simulink model "Navigation_KF_Subsystem_child"  (R2016a)
settings: configuration reference "AR_Drone_ConfigSet" (kept outside this file)
undefined symbols (not defined in the file or in its folder): Accel_Calib_Gain, Accel_Calib_Offset, DiscIntNeverNeededParam, Mag_Calib_Gain_Vector, Mag_Calib_Offset_Vector
libraries: aerolibtransform2 x4, vrlib x4
(part 1 of 2)
settings Model: DataDictionary=ArDroneDataDictionary.sldd  SimulationMode=external  Creator=darenlee  LastModifiedBy=sannem
settings ConfigSetRef: DDName=ArDroneDataDictionary.sldd

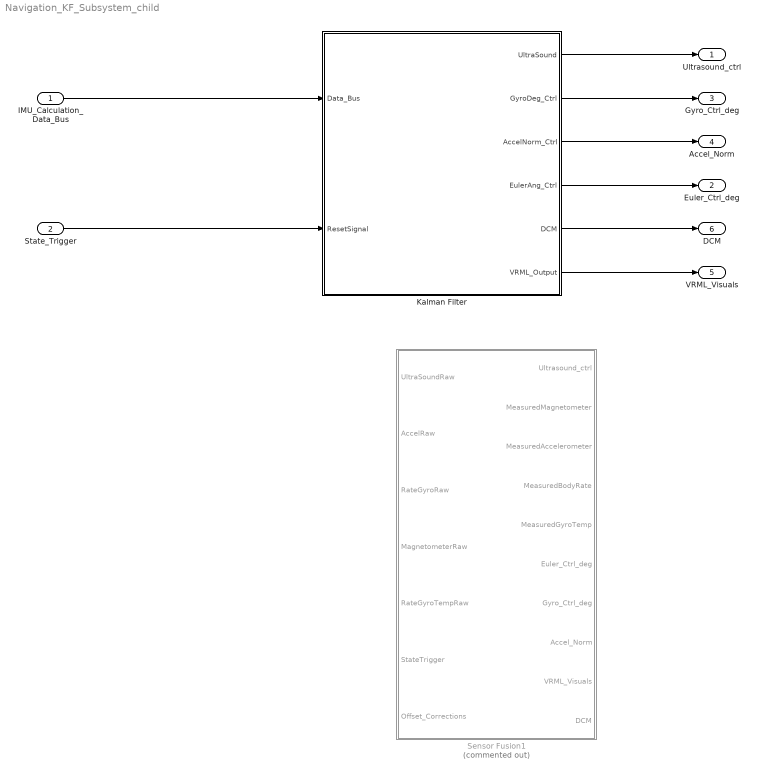
== system Navigation_KF_Subsystem_child ==
  IMU_Calculation_Data_Bus : Inport  OutDataTypeStr=Bus: Measurement_Calculation_Bus
  State_Trigger : Inport  Port=2  OutDataTypeStr=int16
  Kalman Filter : Subsystem
  Sensor Fusion1 : Subsystem  Commented=on
  Ultrasound_ctrl : Outport
  Euler_Ctrl_deg : Outport  Port=2
  Gyro_Ctrl_deg : Outport  Port=3
  Accel_Norm : Outport  Port=4
  VRML_Visuals : Outport  Port=5
  DCM : Outport  Port=6
  wires:
  IMU_Calculation_Data_Bus/1 -> Kalman Filter/1(Data_Bus)
  State_Trigger/1 -> Kalman Filter/2(ResetSignal)
  Kalman Filter/1(UltraSound) -> Ultrasound_ctrl/1
  Kalman Filter/2(GyroDeg_Ctrl) -> Gyro_Ctrl_deg/1
  Kalman Filter/3(AccelNorm_Ctrl) -> Accel_Norm/1
  Kalman Filter/4(EulerAng_Ctrl) -> Euler_Ctrl_deg/1
  Kalman Filter/5(DCM) -> DCM/1
  Kalman Filter/6(VRML_Output) -> VRML_Visuals/1

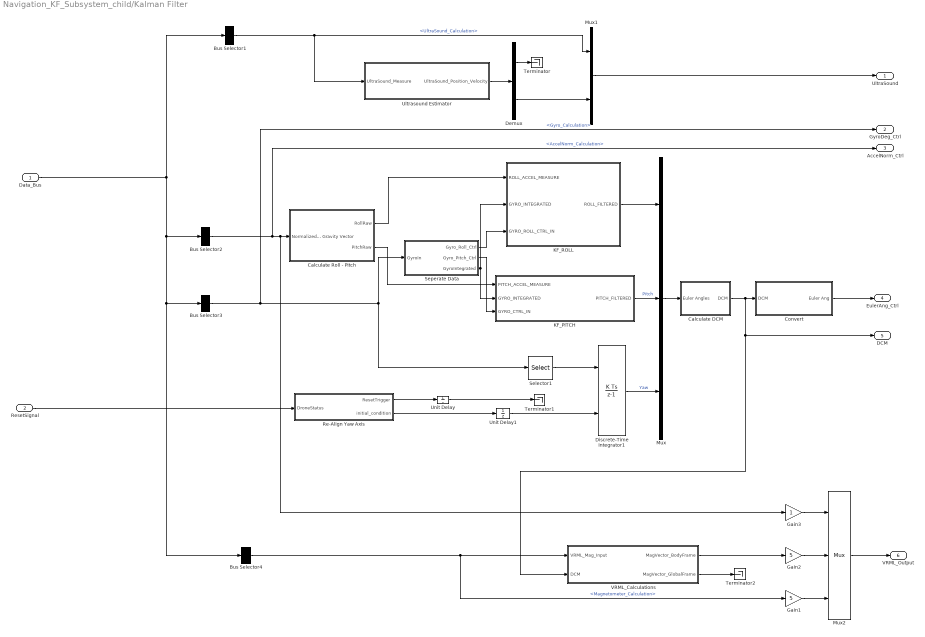
== system Navigation_KF_Subsystem_child/Kalman Filter ==
  Data_Bus : Inport
  ResetSignal : Inport  Port=2
  Bus Selector1 : BusSelector  OutputSignals=UltraSound_Calculation
  Bus Selector2 : BusSelector  OutputSignals=AccelNorm_Calculation
  Bus Selector3 : BusSelector  OutputSignals=Gyro_Calculation
  Bus Selector4 : BusSelector  OutputSignals=Magnetometer_Calculation
  Calculate DCM : Subsystem
  Calculate Roll - Pitch : Subsystem
  Convert : Subsystem
  Demux : Demux  Outputs=2
  Discrete-Time Integrator1 : DiscreteIntegrator  InitialConditionSource=external  SampleTime=1/400  OutDataTypeStr=double  ICPrevOutput=DiscIntNeverNeededParam  ICPrevScaledInput=DiscIntNeverNeededParam
  Gain1 : Gain  Gain=5  OutDataTypeStr=double
  Gain2 : Gain  Gain=5  OutDataTypeStr=double
  Gain3 : Gain  OutDataTypeStr=double
  KF_PITCH : Subsystem
  KF_ROLL : Subsystem
  Mux : Mux  Inputs=3
  Mux1 : Mux  Inputs=2
  Mux2 : Mux  Inputs=3
  Re-Align Yaw Axis : MATLAB Function  TreatAsAtomicUnit=on
  Selector1 : Selector  IndexMode=Zero-based  InputPortWidth=3  IndexOptions=Index vector (dialog)  Indices=[2]  OutputSizes=1
  Seperate Data : Subsystem
  Terminator : Terminator
  Terminator1 : Terminator
  Terminator2 : Terminator
  Ultrasound Estimator : Subsystem
  Unit Delay : UnitDelay  SampleTime=-1
  Unit Delay1 : UnitDelay  SampleTime=-1
  VRML_Calculations : Subsystem
  UltraSound : Outport
  GyroDeg_Ctrl : Outport  Port=2
  AccelNorm_Ctrl : Outport  Port=3
  EulerAng_Ctrl : Outport  Port=4
  DCM : Outport  Port=5
  VRML_Output : Outport  Port=6
  wires:
  Calculate DCM/1(DCM) -> Convert/1(DCM), DCM/1, VRML_Calculations/2(DCM)
  Bus Selector1/1 -> Ultrasound Estimator/1(UltraSound_Measure), Mux1/1  "<UltraSound_Calculation>"
  Unit Delay/1 -> Terminator1/1
  Data_Bus/1 -> Bus Selector4/1, Bus Selector3/1, Bus Selector2/1, Bus Selector1/1
  Re-Align Yaw Axis/1(ResetTrigger) -> Unit Delay/1
  Bus Selector4/1 -> Gain1/1, VRML_Calculations/1(VRML_Mag_Input)  "<Magnetometer_Calculation>"
  Unit Delay1/1 -> Discrete-Time Integrator1/2
  Bus Selector3/1 -> Selector1/1, Seperate Data/1(GyroIn), GyroDeg_Ctrl/1  "<Gyro_Calculation>"
  Calculate Roll - Pitch/2(PitchRaw) -> KF_PITCH/1(PITCH_ACCEL_MEASURE)
  Seperate Data/2(Gyro_Pitch_Ctrl) -> KF_PITCH/3(GYRO_CTRL_IN)
  Discrete-Time Integrator1/1 -> Mux/3  "Yaw"
  Mux/1 -> Calculate DCM/1(Euler Angles)
  Bus Selector2/1 -> Calculate Roll - Pitch/1(Normalized Gravity Vector), Gain3/1, AccelNorm_Ctrl/1  "<AccelNorm_Calculation>"
  Gain3/1 -> Mux2/1
  Ultrasound Estimator/1("UltraSound_Position_Velocity ") -> Demux/1
  KF_PITCH/1(PITCH_FILTERED) -> Mux/2  "Pitch"
  KF_ROLL/1(ROLL_FILTERED) -> Mux/1
  ResetSignal/1 -> Re-Align Yaw Axis/1(DroneStatus)
  Calculate Roll - Pitch/1(RollRaw) -> KF_ROLL/1(ROLL_ACCEL_MEASURE)
  VRML_Calculations/1(MagVector_BodyFrame) -> Gain2/1
  Gain2/1 -> Mux2/2
  Convert/1(Euler Ang) -> EulerAng_Ctrl/1
  Mux2/1 -> VRML_Output/1
  Demux/2 -> Mux1/2
  Gain1/1 -> Mux2/3
  Re-Align Yaw Axis/2(initial_condition) -> Unit Delay1/1
  Mux1/1 -> UltraSound/1
  Seperate Data/3(GyroIntegrated) -> KF_PITCH/2(GYRO_INTEGRATED), KF_ROLL/2(GYRO_INTEGRATED)
  Demux/1 -> Terminator/1
  VRML_Calculations/2(MagVector_GlobalFrame) -> Terminator2/1
  Selector1/1 -> Discrete-Time Integrator1/1
  Seperate Data/1(Gyro_Roll_Ctrl) -> KF_ROLL/3(GYRO_ROLL_CTRL_IN)

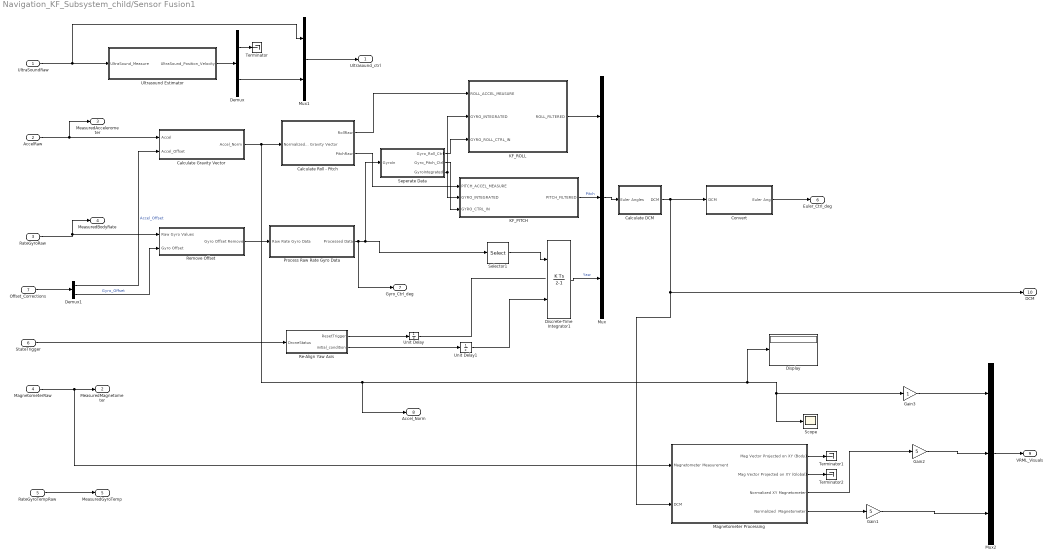
== system Navigation_KF_Subsystem_child/Sensor Fusion1 ==
  UltraSoundRaw : Inport
  AccelRaw : Inport  Port=2
  RateGyroRaw : Inport  Port=3
  MagnetometerRaw : Inport  Port=4
  RateGyroTempRaw : Inport  Port=5
  StateTrigger : Inport  Port=6
  Offset_Corrections : Inport  Port=7
  Calculate DCM : Subsystem
  Calculate Gravity Vector : Subsystem
  Calculate Roll - Pitch : Subsystem
  Convert : Subsystem
  Demux : Demux  Outputs=2
  Demux1 : Demux  Outputs=[2 3]
  Discrete-Time Integrator1 : DiscreteIntegrator  InitialConditionSource=external  SampleTime=1/400  OutDataTypeStr=double  ICPrevOutput=DiscIntNeverNeededParam  ICPrevScaledInput=DiscIntNeverNeededParam
  Display : Display
  Gain1 : Gain  Gain=5  OutDataTypeStr=double
  Gain2 : Gain  Gain=5  OutDataTypeStr=double
  Gain3 : Gain  OutDataTypeStr=double
  KF_PITCH : Subsystem
  KF_ROLL : Subsystem
  Magnetometer Processing : Subsystem  TreatAsAtomicUnit=on
      settings: RTWSystemCode=Inline
  Mux : Mux  Inputs=3
  Mux1 : Mux  Inputs=2
  Mux2 : Mux  Inputs=3
  Process Raw Rate Gyro Data : Subsystem
  Re-Align Yaw Axis : MATLAB Function  TreatAsAtomicUnit=on
  Remove Offset : Subsystem
  Scope : Scope
  Selector1 : Selector  IndexMode=Zero-based  InputPortWidth=3  IndexOptions=Index vector (dialog)  Indices=[2]  OutputSizes=1
  Seperate Data : Subsystem
  Terminator : Terminator
  Terminator1 : Terminator
  Terminator2 : Terminator
  Ultrasound Estimator : Subsystem
  Unit Delay : UnitDelay  SampleTime=-1
  Unit Delay1 : UnitDelay  SampleTime=-1
  Ultrasound_ctrl : Outport
  MeasuredMagnetometer : Outport  Port=2
  MeasuredAccelerometer : Outport  Port=3
  MeasuredBodyRate : Outport  Port=4
  MeasuredGyroTemp : Outport  Port=5
  Euler_Ctrl_deg : Outport  Port=6
  Gyro_Ctrl_deg : Outport  Port=7
  Accel_Norm : Outport  Port=8
  VRML_Visuals : Outport  Port=9
  DCM : Outport  Port=10
  wires:
  Gain1/1 -> Mux2/3
  Gain3/1 -> Mux2/1
  Calculate Roll - Pitch/1(RollRaw) -> KF_ROLL/1(ROLL_ACCEL_MEASURE)
  Calculate Roll - Pitch/2(PitchRaw) -> KF_PITCH/1(PITCH_ACCEL_MEASURE)
  Process Raw Rate Gyro Data/1(Processed Data) -> Selector1/1, Seperate Data/1(GyroIn), Gyro_Ctrl_deg/1
  Mux1/1 -> Ultrasound_ctrl/1
  Ultrasound Estimator/1("UltraSound_Position_Velocity ") -> Demux/1
  Demux/2 -> Mux1/2
  Demux/1 -> Terminator/1
  Discrete-Time Integrator1/1 -> Mux/3  "Yaw"
  KF_PITCH/1(PITCH_FILTERED) -> Mux/2  "Pitch"
  KF_ROLL/1(ROLL_FILTERED) -> Mux/1
  Calculate DCM/1(DCM) -> Magnetometer Processing/2(DCM), DCM/1, Convert/1(DCM)
  Mux/1 -> Calculate DCM/1(Euler Angles)
  Calculate Gravity Vector/1(Accel_Norm) -> Accel_Norm/1, Display/1, Scope/1, Gain3/1, Calculate Roll - Pitch/1(Normalized Gravity Vector)
  Magnetometer Processing/4(Normalized  Magnetometer) -> Gain1/1
  Magnetometer Processing/3(Normalized XY Magnetometer) -> Gain2/1
  Magnetometer Processing/1(Mag Vector Projected on XY (Body)) -> Terminator1/1
  Magnetometer Processing/2(Mag Vector Projected on XY (Global)) -> Terminator2/1
  Remove Offset/1(Gyro Offset Remove) -> Process Raw Rate Gyro Data/1(Raw Rate Gyro Data)
  UltraSoundRaw/1 -> Mux1/1, Ultrasound Estimator/1(UltraSound_Measure)
  MagnetometerRaw/1 -> MeasuredMagnetometer/1, Magnetometer Processing/1(Magnetometer Measurement)
  RateGyroRaw/1 -> MeasuredBodyRate/1, Remove Offset/1(Raw Gyro Values)
  RateGyroTempRaw/1 -> MeasuredGyroTemp/1
  AccelRaw/1 -> MeasuredAccelerometer/1, Calculate Gravity Vector/1(Accel)
  Convert/1(Euler Ang) -> Euler_Ctrl_deg/1
  Re-Align Yaw Axis/1(ResetTrigger) -> Unit Delay/1
  StateTrigger/1 -> Re-Align Yaw Axis/1(DroneStatus)
  Unit Delay/1 -> ?
  Re-Align Yaw Axis/2(initial_condition) -> Unit Delay1/1
  Unit Delay1/1 -> Discrete-Time Integrator1/2
  Selector1/1 -> Discrete-Time Integrator1/1
  Seperate Data/1(Gyro_Roll_Ctrl) -> KF_ROLL/3(GYRO_ROLL_CTRL_IN)
  Seperate Data/2(Gyro_Pitch_Ctrl) -> KF_PITCH/3(GYRO_CTRL_IN)
  Seperate Data/3(GyroIntegrated) -> KF_PITCH/2(GYRO_INTEGRATED), KF_ROLL/2(GYRO_INTEGRATED)
  Offset_Corrections/1 -> Demux1/1
  Demux1/1 -> Calculate Gravity Vector/2(Accel_Offset)  "Accel_Offset"
  Demux1/2 -> Remove Offset/2(Gyro Offset)  "Gyro_Offset"
  Gain2/1 -> Mux2/2
  Mux2/1 -> VRML_Visuals/1

== system Navigation_KF_Subsystem_child/Kalman Filter/Calculate DCM ==
  Euler Angles : Inport
  Change Sign : Gain  Gain=-1
  Rad2deg : Gain  Gain=pi/180
  Rotation Angles to Direction Cosine Matrix : aerolibtransform2/Rotation Angles to Direction Cosine Matrix  rotationOrder=XYZ
  DCM : Outport
  wires:
  Euler Angles/1 -> Change Sign/1
  Rotation Angles to Direction Cosine Matrix/1 -> DCM/1
  Change Sign/1 -> Rad2deg/1
  Rad2deg/1 -> Rotation Angles to Direction Cosine Matrix/1

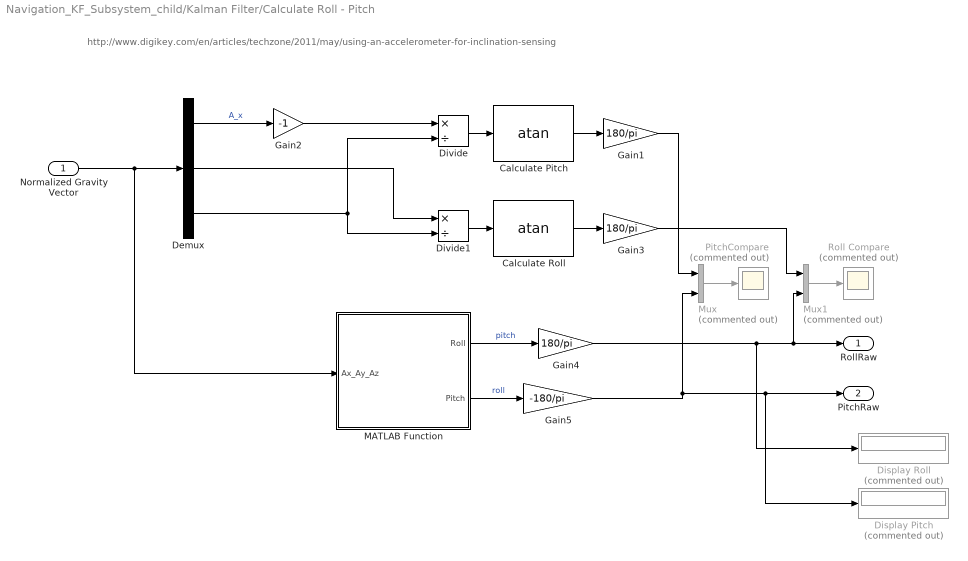
== system Navigation_KF_Subsystem_child/Kalman Filter/Calculate Roll - Pitch ==
  note: http://www.digikey.com/en/articles/techzone/2011/may/using-an-accelerometer-for-inclination-sensing
  Normalized Gravity Vector : Inport
  Calculate Pitch : Trigonometry  Operator=atan
  Calculate Roll : Trigonometry  Operator=atan
  Demux : Demux  Outputs=3
  Display Pitch : Display  Commented=on
  Display Roll : Display  Commented=on
  Divide : Product  Inputs=*/
  Divide1 : Product  Inputs=*/
  Gain1 : Gain  Gain=180/pi
  Gain2 : Gain  Gain=-1
  Gain3 : Gain  Gain=180/pi
  Gain4 : Gain  Gain=180/pi
  Gain5 : Gain  Gain=-180/pi
  MATLAB Function : MATLAB Function  TreatAsAtomicUnit=on
  Mux : Mux  Commented=on  Inputs=2
  Mux1 : Mux  Commented=on  Inputs=2
  PitchCompare : Scope  Commented=on
  Roll Compare : Scope  Commented=on
  RollRaw : Outport
  PitchRaw : Outport  Port=2
  wires:
  Divide/1 -> Calculate Pitch/1
  Gain2/1 -> Divide/1
  Demux/2 -> Divide1/1
  Divide1/1 -> Calculate Roll/1
  Calculate Pitch/1 -> Gain1/1
  Demux/3 -> Divide/2, Divide1/2
  Calculate Roll/1 -> Gain3/1
  Demux/1 -> Gain2/1  "A_x"
  Normalized Gravity Vector/1 -> MATLAB Function/1(Ax_Ay_Az), Demux/1
  MATLAB Function/1(Roll) -> Gain4/1  "pitch"
  MATLAB Function/2(Pitch) -> Gain5/1  "roll"
  Gain4/1 -> RollRaw/1, Mux1/2, Display Roll/1
  Gain1/1 -> Mux/1
  Mux/1 -> PitchCompare/1
  Gain5/1 -> PitchRaw/1, Display Pitch/1, Mux/2
  Gain3/1 -> Mux1/1
  Mux1/1 -> Roll Compare/1

== system Navigation_KF_Subsystem_child/Kalman Filter/Convert ==
  note: This susystem might be removed in the future
      | This is done to be consistent with how the drone's SL3D block
      | functions
  DCM : Inport
  DCM to Euler Angles : Subsystem
  Gain : Gain  Gain=180/pi
  Euler Ang : Outport
  wires:
  DCM to Euler Angles/1(Euler_Block) -> Gain/1
  Gain/1 -> Euler Ang/1
  DCM/1 -> DCM to Euler Angles/1(DCM)

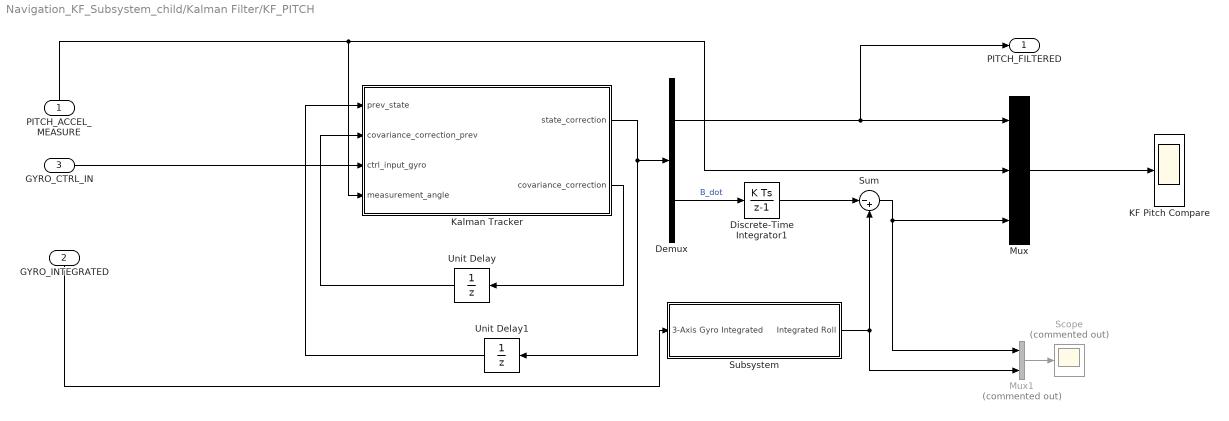
== system Navigation_KF_Subsystem_child/Kalman Filter/KF_PITCH ==
  PITCH_ACCEL_MEASURE : Inport
  GYRO_INTEGRATED : Inport  Port=2
  GYRO_CTRL_IN : Inport  Port=3
  Demux : Demux  Outputs=2
  Discrete-Time Integrator1 : DiscreteIntegrator  SampleTime=1/400  ICPrevOutput=DiscIntNeverNeededParam  ICPrevScaledInput=DiscIntNeverNeededParam
  KF Pitch Compare : Scope
  Kalman Tracker : MATLAB Function  TreatAsAtomicUnit=on
  Mux : Mux  Inputs=3
  Mux1 : Mux  Commented=on  Inputs=2
  Scope : Scope  Commented=on
  Subsystem : Subsystem
  Sum : Sum  Inputs=|-+
  Unit Delay : UnitDelay  InitialCondition=eye(2)  SampleTime=-1
  Unit Delay1 : UnitDelay  InitialCondition=[0 0]'  SampleTime=-1
  PITCH_FILTERED : Outport
  wires:
  Mux1/1 -> Scope/1
  Discrete-Time Integrator1/1 -> Sum/1
  Demux/2 -> Discrete-Time Integrator1/1  "B_dot"
  Sum/1 -> Mux1/1, Mux/3
  Subsystem/1(Integrated Roll) -> Mux1/2, Sum/2
  Kalman Tracker/2(covariance_correction) -> Unit Delay/1
  Demux/1 -> PITCH_FILTERED/1, Mux/1
  Kalman Tracker/1(state_correction) -> Unit Delay1/1, Demux/1
  Mux/1 -> KF Pitch Compare/1
  Unit Delay1/1 -> Kalman Tracker/1(prev_state)
  GYRO_CTRL_IN/1 -> Kalman Tracker/3(ctrl_input_gyro)
  Unit Delay/1 -> Kalman Tracker/2(covariance_correction_prev)
  GYRO_INTEGRATED/1 -> Subsystem/1(3-Axis Gyro Integrated)
  PITCH_ACCEL_MEASURE/1 -> Kalman Tracker/4(measurement_angle), Mux/2

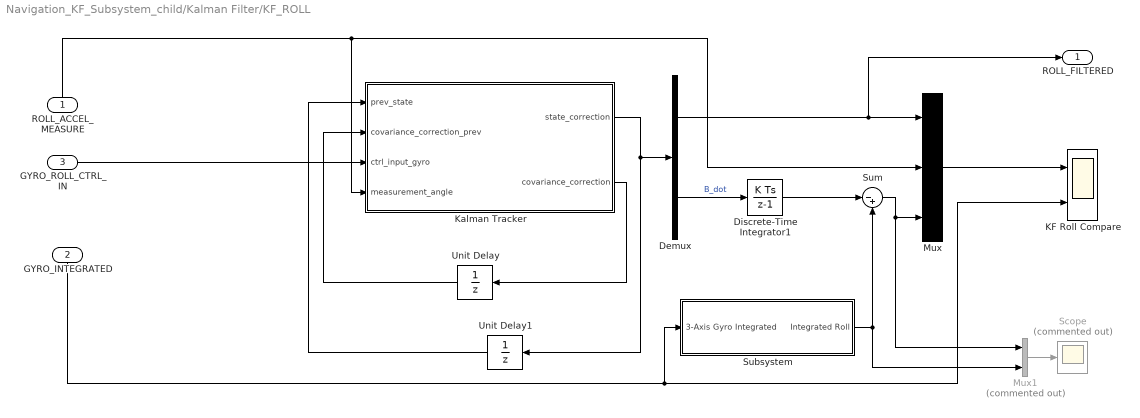
== system Navigation_KF_Subsystem_child/Kalman Filter/KF_ROLL ==
  ROLL_ACCEL_MEASURE : Inport
  GYRO_INTEGRATED : Inport  Port=2
  GYRO_ROLL_CTRL_IN : Inport  Port=3
  Demux : Demux  Outputs=2
  Discrete-Time Integrator1 : DiscreteIntegrator  SampleTime=1/400  ICPrevOutput=DiscIntNeverNeededParam  ICPrevScaledInput=DiscIntNeverNeededParam
  KF Roll Compare : Scope  NumInputPorts=2
  Kalman Tracker : MATLAB Function  TreatAsAtomicUnit=on
  Mux : Mux  Inputs=3
  Mux1 : Mux  Commented=on  Inputs=2
  Scope : Scope  Commented=on
  Subsystem : Subsystem
  Sum : Sum  Inputs=|-+
  Unit Delay : UnitDelay  InitialCondition=eye(2)  SampleTime=-1
  Unit Delay1 : UnitDelay  InitialCondition=[0 0]'  SampleTime=-1
  ROLL_FILTERED : Outport
  wires:
  Mux1/1 -> Scope/1
  Discrete-Time Integrator1/1 -> Sum/1
  Demux/2 -> Discrete-Time Integrator1/1  "B_dot"
  Sum/1 -> Mux1/1, Mux/3
  Subsystem/1(Integrated Roll) -> Mux1/2, Sum/2
  Kalman Tracker/2(covariance_correction) -> Unit Delay/1
  Kalman Tracker/1(state_correction) -> Unit Delay1/1, Demux/1
  Mux/1 -> KF Roll Compare/1
  Unit Delay1/1 -> Kalman Tracker/1(prev_state)
  GYRO_ROLL_CTRL_IN/1 -> Kalman Tracker/3(ctrl_input_gyro)
  Unit Delay/1 -> Kalman Tracker/2(covariance_correction_prev)
  GYRO_INTEGRATED/1 -> KF Roll Compare/2, Subsystem/1(3-Axis Gyro Integrated)
  ROLL_ACCEL_MEASURE/1 -> Kalman Tracker/4(measurement_angle), Mux/2
  Demux/1 -> ROLL_FILTERED/1, Mux/1

== system Navigation_KF_Subsystem_child/Kalman Filter/Seperate Data ==
  GyroIn : Inport
  Demux1 : Demux  Outputs=[1 1]
  Discrete-Time Integrator1 : DiscreteIntegrator  SampleTime=1/400  ICPrevOutput=DiscIntNeverNeededParam  ICPrevScaledInput=DiscIntNeverNeededParam
  Selector2 : Selector  IndexMode=Zero-based  InputPortWidth=3  IndexOptions=Index vector (dialog)  Indices=[0 1]  OutputSizes=1
  Gyro_Roll_Ctrl : Outport
  Gyro_Pitch_Ctrl : Outport  Port=2
  GyroIntegrated : Outport  Port=3
  wires:
  GyroIn/1 -> Discrete-Time Integrator1/1, Selector2/1
  Demux1/1 -> Gyro_Roll_Ctrl/1  "GYRO_X"
  Demux1/2 -> Gyro_Pitch_Ctrl/1  "GYRO_Y"
  Selector2/1 -> Demux1/1
  Discrete-Time Integrator1/1 -> GyroIntegrated/1

== system Navigation_KF_Subsystem_child/Kalman Filter/Ultrasound Estimator ==
  UltraSound_Measure : Inport
  Kalman Tracker : MATLAB Function  TreatAsAtomicUnit=on
  Unit Delay1 : UnitDelay  InitialCondition=[0 0 ]  SampleTime=-1
  Unit Delay2 : UnitDelay  InitialCondition=eye(2)  SampleTime=-1
  "UltraSound_Position_Velocity " : Outport
  wires:
  Kalman Tracker/2(covariance_correction) -> Unit Delay2/1
  Kalman Tracker/1(state_correction) -> Unit Delay1/1
  UltraSound_Measure/1 -> Kalman Tracker/1(UltraSoundMeasure)
  Unit Delay2/1 -> Kalman Tracker/2(covariance_correction_input)
  Unit Delay1/1 -> "UltraSound_Position_Velocity "/1, Kalman Tracker/3(state_correction_input)

== system Navigation_KF_Subsystem_child/Kalman Filter/VRML_Calculations ==
  VRML_Mag_Input : Inport
  DCM : Inport  Port=2
  Magnetometer Heading Calculation : Subsystem
  Normalize Vector1 : vrlib/Utilities/Normalize Vector  maxzero=0
  Re-align X-axis : Subsystem
  MagVector_BodyFrame : Outport
  MagVector_GlobalFrame : Outport  Port=2
  wires:
  VRML_Mag_Input/1 -> Re-align X-axis/1(MagVector)
  Re-align X-axis/1(MagVectorOut) -> Magnetometer Heading Calculation/1(MagVector)
  Magnetometer Heading Calculation/1(Projected Mag Vector (body frame)) -> Normalize Vector1/1
  Normalize Vector1/1 -> MagVector_BodyFrame/1
  DCM/1 -> Magnetometer Heading Calculation/2(DCM)
  Magnetometer Heading Calculation/2(Projected Mag Vector (global frame)) -> MagVector_GlobalFrame/1

== system Navigation_KF_Subsystem_child/Sensor Fusion1/Calculate DCM ==
  Euler Angles : Inport
  Change Sign : Gain  Gain=-1
  Rad2deg : Gain  Gain=pi/180
  Rotation Angles to Direction Cosine Matrix : aerolibtransform2/Rotation Angles to Direction Cosine Matrix  rotationOrder=XYZ
  DCM : Outport
  wires:
  Euler Angles/1 -> Change Sign/1
  Rotation Angles to Direction Cosine Matrix/1 -> DCM/1
  Change Sign/1 -> Rad2deg/1
  Rad2deg/1 -> Rotation Angles to Direction Cosine Matrix/1

== system Navigation_KF_Subsystem_child/Sensor Fusion1/Calculate Gravity Vector ==
  Accel : Inport
  Accel_Offset : Inport  Port=2
  Accelerometer Neutral Gain and Offset : Subsystem
  Calibration_GainOffset : Subsystem
  Compare Calibration : Scope  NumInputPorts=2
  Compare Filter : Scope  NumInputPorts=2
  Compare Offset : Scope  NumInputPorts=2
  InitialCondition_Offset : Subsystem
  Low Pass Filter : Subsystem
  Normalize Vector : vrlib/Utilities/Normalize Vector  maxzero=0
  Accel_Norm : Outport
  wires:
  Normalize Vector/1 -> Accel_Norm/1
  Accel/1 -> Accelerometer Neutral Gain and Offset/1(Raw Accel Data)
  InitialCondition_Offset/1(Post) -> Compare Offset/1, Compare Filter/2, Low Pass Filter/1(Offset Accel)
  Low Pass Filter/1(Filtered Accel) -> Compare Filter/1, Normalize Vector/1
  Calibration_GainOffset/1(Post) -> InitialCondition_Offset/1(Pre), Compare Calibration/1, Compare Offset/2
  Accelerometer Neutral Gain and Offset/1(Processed Accel Data) -> Calibration_GainOffset/1(Pre), Compare Calibration/2
  Accel_Offset/1 -> InitialCondition_Offset/2(Accel_Offset)

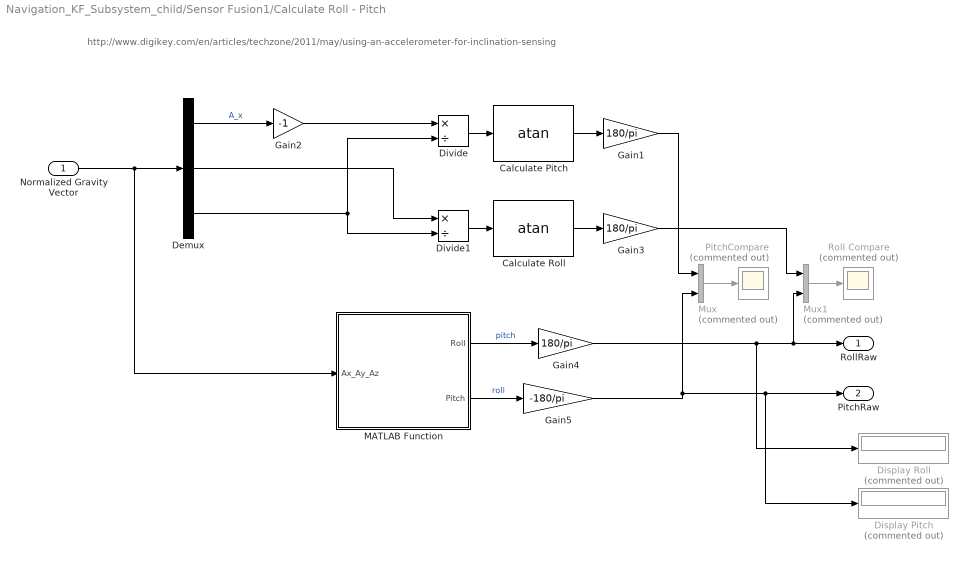
== system Navigation_KF_Subsystem_child/Sensor Fusion1/Calculate Roll - Pitch ==
  note: http://www.digikey.com/en/articles/techzone/2011/may/using-an-accelerometer-for-inclination-sensing
  Normalized Gravity Vector : Inport
  Calculate Pitch : Trigonometry  Operator=atan
  Calculate Roll : Trigonometry  Operator=atan
  Demux : Demux  Outputs=3
  Display Pitch : Display  Commented=on
  Display Roll : Display  Commented=on
  Divide : Product  Inputs=*/
  Divide1 : Product  Inputs=*/
  Gain1 : Gain  Gain=180/pi
  Gain2 : Gain  Gain=-1
  Gain3 : Gain  Gain=180/pi
  Gain4 : Gain  Gain=180/pi
  Gain5 : Gain  Gain=-180/pi
  MATLAB Function : MATLAB Function  TreatAsAtomicUnit=on
  Mux : Mux  Commented=on  Inputs=2
  Mux1 : Mux  Commented=on  Inputs=2
  PitchCompare : Scope  Commented=on
  Roll Compare : Scope  Commented=on
  RollRaw : Outport
  PitchRaw : Outport  Port=2
  wires:
  Divide/1 -> Calculate Pitch/1
  Gain2/1 -> Divide/1
  Demux/2 -> Divide1/1
  Divide1/1 -> Calculate Roll/1
  Calculate Pitch/1 -> Gain1/1
  Demux/3 -> Divide/2, Divide1/2
  Calculate Roll/1 -> Gain3/1
  Demux/1 -> Gain2/1  "A_x"
  Normalized Gravity Vector/1 -> MATLAB Function/1(Ax_Ay_Az), Demux/1
  MATLAB Function/1(Roll) -> Gain4/1  "pitch"
  MATLAB Function/2(Pitch) -> Gain5/1  "roll"
  Gain4/1 -> RollRaw/1, Mux1/2, Display Roll/1
  Gain1/1 -> Mux/1
  Mux/1 -> PitchCompare/1
  Gain5/1 -> PitchRaw/1, Display Pitch/1, Mux/2
  Gain3/1 -> Mux1/1
  Mux1/1 -> Roll Compare/1

== system Navigation_KF_Subsystem_child/Sensor Fusion1/Convert ==
  note: This susystem might be removed in the future
      | This is done to be consistent with how the drone's SL3D block
      | functions
  DCM : Inport
  DCM to Euler Angles : Subsystem
  Gain : Gain  Gain=180/pi
  Euler Ang : Outport
  wires:
  DCM to Euler Angles/1(Euler_Block) -> Gain/1
  Gain/1 -> Euler Ang/1
  DCM/1 -> DCM to Euler Angles/1(DCM)

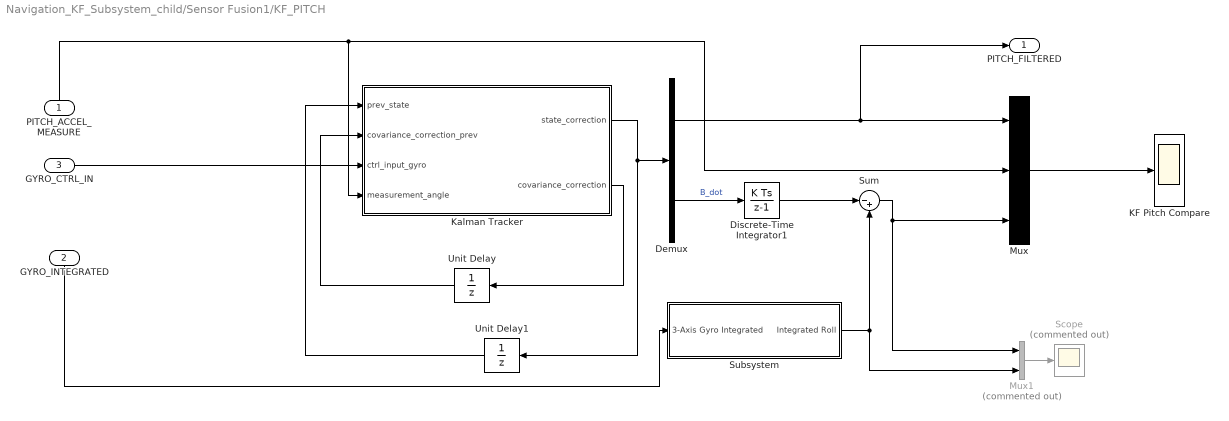
== system Navigation_KF_Subsystem_child/Sensor Fusion1/KF_PITCH ==
  PITCH_ACCEL_MEASURE : Inport
  GYRO_INTEGRATED : Inport  Port=2
  GYRO_CTRL_IN : Inport  Port=3
  Demux : Demux  Outputs=2
  Discrete-Time Integrator1 : DiscreteIntegrator  SampleTime=1/400  ICPrevOutput=DiscIntNeverNeededParam  ICPrevScaledInput=DiscIntNeverNeededParam
  KF Pitch Compare : Scope
  Kalman Tracker : MATLAB Function  TreatAsAtomicUnit=on
  Mux : Mux  Inputs=3
  Mux1 : Mux  Commented=on  Inputs=2
  Scope : Scope  Commented=on
  Subsystem : Subsystem
  Sum : Sum  Inputs=|-+
  Unit Delay : UnitDelay  InitialCondition=eye(2)  SampleTime=-1
  Unit Delay1 : UnitDelay  InitialCondition=[0 0]'  SampleTime=-1
  PITCH_FILTERED : Outport
  wires:
  Mux1/1 -> Scope/1
  Discrete-Time Integrator1/1 -> Sum/1
  Demux/2 -> Discrete-Time Integrator1/1  "B_dot"
  Sum/1 -> Mux1/1, Mux/3
  Subsystem/1(Integrated Roll) -> Mux1/2, Sum/2
  Kalman Tracker/2(covariance_correction) -> Unit Delay/1
  Demux/1 -> PITCH_FILTERED/1, Mux/1
  Kalman Tracker/1(state_correction) -> Unit Delay1/1, Demux/1
  Mux/1 -> KF Pitch Compare/1
  Unit Delay1/1 -> Kalman Tracker/1(prev_state)
  GYRO_CTRL_IN/1 -> Kalman Tracker/3(ctrl_input_gyro)
  Unit Delay/1 -> Kalman Tracker/2(covariance_correction_prev)
  GYRO_INTEGRATED/1 -> Subsystem/1(3-Axis Gyro Integrated)
  PITCH_ACCEL_MEASURE/1 -> Kalman Tracker/4(measurement_angle), Mux/2

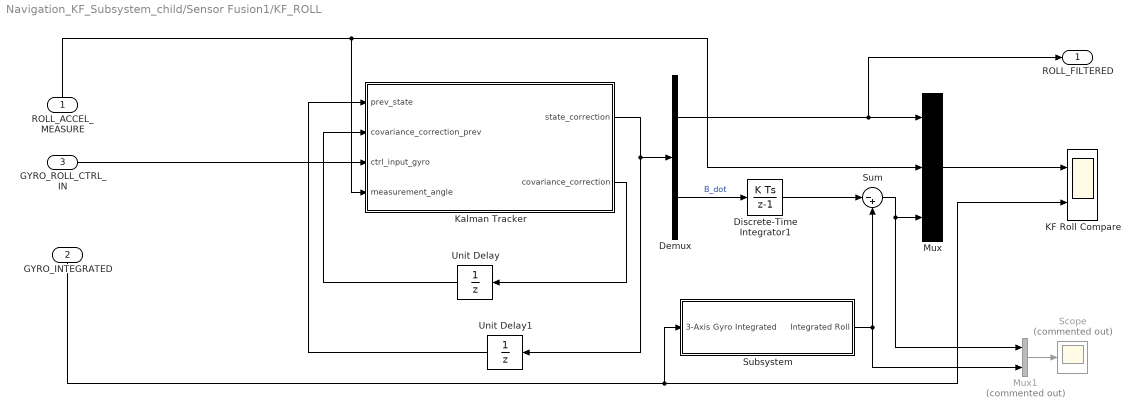
== system Navigation_KF_Subsystem_child/Sensor Fusion1/KF_ROLL ==
  ROLL_ACCEL_MEASURE : Inport
  GYRO_INTEGRATED : Inport  Port=2
  GYRO_ROLL_CTRL_IN : Inport  Port=3
  Demux : Demux  Outputs=2
  Discrete-Time Integrator1 : DiscreteIntegrator  SampleTime=1/400  ICPrevOutput=DiscIntNeverNeededParam  ICPrevScaledInput=DiscIntNeverNeededParam
  KF Roll Compare : Scope  NumInputPorts=2
  Kalman Tracker : MATLAB Function  TreatAsAtomicUnit=on
  Mux : Mux  Inputs=3
  Mux1 : Mux  Commented=on  Inputs=2
  Scope : Scope  Commented=on
  Subsystem : Subsystem
  Sum : Sum  Inputs=|-+
  Unit Delay : UnitDelay  InitialCondition=eye(2)  SampleTime=-1
  Unit Delay1 : UnitDelay  InitialCondition=[0 0]'  SampleTime=-1
  ROLL_FILTERED : Outport
  wires:
  Mux1/1 -> Scope/1
  Discrete-Time Integrator1/1 -> Sum/1
  Demux/2 -> Discrete-Time Integrator1/1  "B_dot"
  Sum/1 -> Mux1/1, Mux/3
  Subsystem/1(Integrated Roll) -> Mux1/2, Sum/2
  Kalman Tracker/2(covariance_correction) -> Unit Delay/1
  Kalman Tracker/1(state_correction) -> Unit Delay1/1, Demux/1
  Mux/1 -> KF Roll Compare/1
  Unit Delay1/1 -> Kalman Tracker/1(prev_state)
  GYRO_ROLL_CTRL_IN/1 -> Kalman Tracker/3(ctrl_input_gyro)
  Unit Delay/1 -> Kalman Tracker/2(covariance_correction_prev)
  GYRO_INTEGRATED/1 -> KF Roll Compare/2, Subsystem/1(3-Axis Gyro Integrated)
  ROLL_ACCEL_MEASURE/1 -> Kalman Tracker/4(measurement_angle), Mux/2
  Demux/1 -> ROLL_FILTERED/1, Mux/1

== system Navigation_KF_Subsystem_child/Sensor Fusion1/Magnetometer Processing ==
  Magnetometer Measurement : Inport
  DCM : Inport  Port=2
  Magnetometer Heading Calculation : Subsystem
  Normalize Vector : vrlib/Utilities/Normalize Vector  maxzero=0
  Normalize Vector1 : vrlib/Utilities/Normalize Vector  maxzero=0
  Process Raw Mag Data : Subsystem  Variant=on  OverrideUsingVariant=TempVariantA
  Re-align X-axis : Subsystem
  Mag Vector Projected on XY (Body) : Outport
  Mag Vector Projected on XY (Global) : Outport  Port=2
  Normalized XY Magnetometer : Outport  Port=3
  Normalized  Magnetometer : Outport  Port=4
  wires:
  Magnetometer Heading Calculation/2(Projected Mag Vector (global frame)) -> Mag Vector Projected on XY (Global)/1
  Normalize Vector/1 -> Normalized  Magnetometer/1, Re-align X-axis/1(MagVector)
  Process Raw Mag Data/1(MagVector) -> Normalize Vector/1
  Re-align X-axis/1(MagVectorOut) -> Magnetometer Heading Calculation/1(MagVector)
  Magnetometer Measurement/1 -> Process Raw Mag Data/1(Magnetometer)
  Magnetometer Heading Calculation/1(Projected Mag Vector (body frame)) -> Normalize Vector1/1
  DCM/1 -> Magnetometer Heading Calculation/2(DCM)
  Normalize Vector1/1 -> Normalized XY Magnetometer/1, Mag Vector Projected on XY (Body)/1

== system Navigation_KF_Subsystem_child/Sensor Fusion1/Process Raw Rate Gyro Data ==
  note: const float Sensitivity[ 3 ] = { 0.0609 , 0.0609 , 0.0609 } ;
      | const float Neutral[ 3 ] = { 0.0 , 0.0 , 0.0 } ;
      | const int16_t Offset[ 3 ] = { - 73 , 14 , - 13 } ;
      | const int16_t Noises[ 3 ] = { 35 , 35 , 15 } ;
      |
      | int16_t vRaws[ 3 ] = {
      | Navdata :: IMU :: Gyroscope :: getRawX (),
      | Navdata :: IMU :: Gyroscope :: getRawY (),
      | Navdata :: IMU :: Gyroscope :: getRawZ ()
      | } ;
      |
      | gyroscope[i] = vRaws[i] * Gyroscope :: Sensitivity[i] * M_PI / 180.0 ;
  Raw Rate Gyro Data : Inport
  Gain : Gain  Gain=[0.0609, 0.0609, 0.0609]  ParamDataTypeStr=double
  Processed Data : Outport
  wires:
  Raw Rate Gyro Data/1 -> Gain/1
  Gain/1 -> Processed Data/1

== system Navigation_KF_Subsystem_child/Sensor Fusion1/Remove Offset ==
  Raw Gyro Values : Inport
  Gyro Offset : Inport  Port=2
  BeforeAfter : Scope
  Demux : Demux  Outputs=3
  Demux1 : Demux  Outputs=3
  Display : Display
  Mux : Mux  Inputs=2
  Mux1 : Mux  Inputs=3
  Sum : Sum  Inputs=|+-
  Sum1 : Sum  Inputs=|+-
  Sum2 : Sum  Inputs=|+-
  Gyro Offset Remove : Outport
  tag scope: GyroOffset_Tag=global
  wires:
  Sum/1 -> Mux1/1
  Sum2/1 -> Mux1/3
  Demux/3 -> Sum2/1
  Sum1/1 -> Mux1/2
  Demux/1 -> Sum/1
  Demux/2 -> Sum1/1
  Demux1/1 -> Sum/2
  Demux1/2 -> Sum1/2
  Demux1/3 -> Sum2/2
  Mux1/1 -> Mux/2, Display/1, Gyro Offset Remove/1
  Gyro Offset/1 -> Demux1/1
  Raw Gyro Values/1 -> [GyroOffset_Tag], Mux/1, Demux/1
  Mux/1 -> BeforeAfter/1

== system Navigation_KF_Subsystem_child/Sensor Fusion1/Seperate Data ==
  GyroIn : Inport
  Demux1 : Demux  Outputs=[1 1]
  Discrete-Time Integrator1 : DiscreteIntegrator  SampleTime=1/400  ICPrevOutput=DiscIntNeverNeededParam  ICPrevScaledInput=DiscIntNeverNeededParam
  Selector2 : Selector  IndexMode=Zero-based  InputPortWidth=3  IndexOptions=Index vector (dialog)  Indices=[0 1]  OutputSizes=1
  Gyro_Roll_Ctrl : Outport
  Gyro_Pitch_Ctrl : Outport  Port=2
  GyroIntegrated : Outport  Port=3
  wires:
  GyroIn/1 -> Discrete-Time Integrator1/1, Selector2/1
  Demux1/1 -> Gyro_Roll_Ctrl/1  "GYRO_X"
  Demux1/2 -> Gyro_Pitch_Ctrl/1  "GYRO_Y"
  Selector2/1 -> Demux1/1
  Discrete-Time Integrator1/1 -> GyroIntegrated/1

== system Navigation_KF_Subsystem_child/Sensor Fusion1/Ultrasound Estimator ==
  UltraSound_Measure : Inport
  Kalman Tracker : MATLAB Function  TreatAsAtomicUnit=on
  Unit Delay1 : UnitDelay  InitialCondition=[0 0 ]  SampleTime=-1
  Unit Delay2 : UnitDelay  InitialCondition=eye(2)  SampleTime=-1
  "UltraSound_Position_Velocity " : Outport
  wires:
  Kalman Tracker/2(covariance_correction) -> Unit Delay2/1
  Kalman Tracker/1(state_correction) -> Unit Delay1/1
  UltraSound_Measure/1 -> Kalman Tracker/1(UltraSoundMeasure)
  Unit Delay2/1 -> Kalman Tracker/2(covariance_correction_input)
  Unit Delay1/1 -> "UltraSound_Position_Velocity "/1, Kalman Tracker/3(state_correction_input)

== system Navigation_KF_Subsystem_child/Kalman Filter/Convert/DCM to Euler Angles ==
  note: Euler Rotation Order:
      | With the camera facing towards you
      | ______________
      |       Camera          |
      | 1                    2    |
      |                             |
      | 3                    4    |
      | ______________|
      |
      | Rotation
      |
      | Roll+ , increase 2+4
      | Roll - , increase 1 3
      |
      | Pitch+ , increaes 1+2
      | Pitch- , increase 3+4
  DCM : Inport
  Constant2 : Constant  Value=[1 0 0]
  Direction Cosine Matrix to Rotation Angles : aerolibtransform2/Direction Cosine Matrix to Rotation Angles  rotationOrder=XYZ  lim=Default
      settings: AttributesFormatString=Rotation Order: %<rotationOrder>
  EulerAnglesCalculation : Subsystem  TreatAsAtomicUnit=on
  Product : Product  Multiplication=Matrix(*)
  Terminator1 : Terminator
  Terminator3 : Terminator
  Euler_Block : Outport
  wires:
  DCM/1 -> Direction Cosine Matrix to Rotation Angles/1, Product/1, EulerAnglesCalculation/1(DCM)
  Direction Cosine Matrix to Rotation Angles/1 -> Euler_Block/1
  Constant2/1 -> Product/2
  EulerAnglesCalculation/1(Euler Angles) -> Terminator3/1
  Product/1 -> Terminator1/1

== system Navigation_KF_Subsystem_child/Kalman Filter/KF_PITCH/Subsystem ==
  3-Axis Gyro Integrated : Inport
  Demux2 : Demux  Outputs=3
  Integrated Roll : Outport
  wires:
  Demux2/2 -> Integrated Roll/1  "Roll Axis"
  3-Axis Gyro Integrated/1 -> Demux2/1

== system Navigation_KF_Subsystem_child/Kalman Filter/KF_ROLL/Subsystem ==
  3-Axis Gyro Integrated : Inport
  Demux2 : Demux  Outputs=3
  Integrated Roll : Outport
  wires:
  Demux2/1 -> Integrated Roll/1  "Roll Axis"
  3-Axis Gyro Integrated/1 -> Demux2/1

== system Navigation_KF_Subsystem_child/Kalman Filter/VRML_Calculations/Magnetometer Heading Calculation ==
  MagVector : Inport
  DCM : Inport  Port=2
  Compensate for Magnetic Declination (~60 degrees in Boston)_ : MATLAB Function  Commented=through  TreatAsAtomicUnit=on
  Compensate for Magnetic Declination (~67 degrees in Boston)_2 : MATLAB Function  TreatAsAtomicUnit=on
  EnlargeVectorAgain : Gain  Commented=through  Gain=3
  Transform MagVector from Body Frame to World Frame : Product  Multiplication=Matrix(*)
  Transform compensated magnetic vector into the  body frame : Product  Multiplication=Matrix(*)
  Transpose2 : Math  Operator=transpose  SaturateOnIntegerOverflow=on
  deg : Constant  Value=67
  Projected Mag Vector (body frame) : Outport
  Projected Mag Vector (global frame) : Outport  Port=2
  wires:
  MagVector/1 -> EnlargeVectorAgain/1
  Transform compensated magnetic vector into the  body frame/1 -> Projected Mag Vector (body frame)/1
  DCM/1 -> Transpose2/1, Transform MagVector from Body Frame to World Frame/1
  EnlargeVectorAgain/1 -> Transform MagVector from Body Frame to World Frame/2
  Transpose2/1 -> Transform compensated magnetic vector into the  body frame/1
  Transform MagVector from Body Frame to World Frame/1 -> Compensate for Magnetic Declination (~60 degrees in Boston)_/1(vector_in)
  Compensate for Magnetic Declination (~60 degrees in Boston)_/1(y) -> Compensate for Magnetic Declination (~67 degrees in Boston)_2/1(vector_in)
  Compensate for Magnetic Declination (~67 degrees in Boston)_2/1(y) -> Transform compensated magnetic vector into the  body frame/2, Projected Mag Vector (global frame)/1
  deg/1 -> Compensate for Magnetic Declination (~67 degrees in Boston)_2/2(declination_ang)

== system Navigation_KF_Subsystem_child/Kalman Filter/VRML_Calculations/Re-align X-axis ==
  MagVector : Inport
  Demux1 : Demux  Outputs=3
  Gain : Gain
  Gain1 : Gain  Gain=-1
  Gain2 : Gain
  Mux2 : Mux  Inputs=3
  MagVectorOut : Outport
  wires:
  Mux2/1 -> MagVectorOut/1
  Demux1/1 -> Gain1/1
  Demux1/2 -> Gain2/1
  Demux1/3 -> Gain/1
  Gain1/1 -> Mux2/1
  Gain2/1 -> Mux2/2
  Gain/1 -> Mux2/3
  MagVector/1 -> Demux1/1

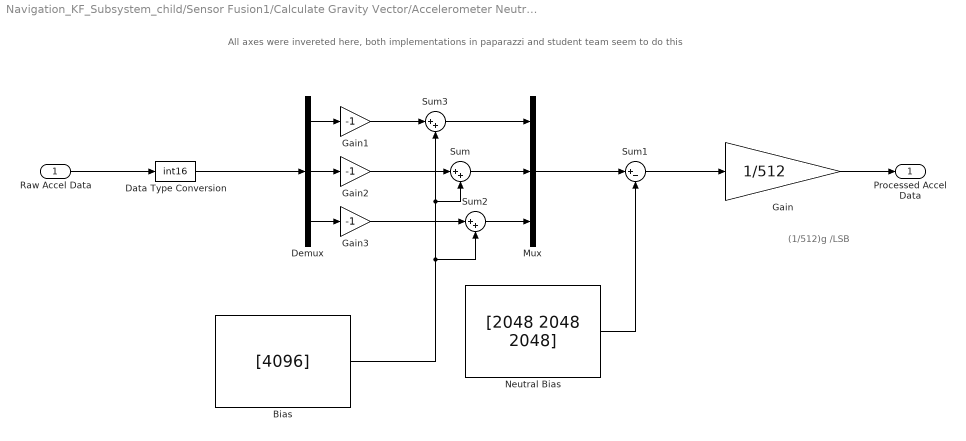
== system Navigation_KF_Subsystem_child/Sensor Fusion1/Calculate Gravity Vector/Accelerometer Neutral Gain and Offset ==
  note: All axes were invereted here, both implementations in paparazzi and student team seem to do this
  note: (1/512)g /LSB
  Raw Accel Data : Inport
  Bias : Constant  Value=[4096]
  Data Type Conversion : DataTypeConversion  OutDataTypeStr=int16
  Demux : Demux  Outputs=3
  Gain : Gain  Gain=1/512
  Gain1 : Gain  Gain=-1  OutDataTypeStr=double
  Gain2 : Gain  Gain=-1  OutDataTypeStr=double
  Gain3 : Gain  Gain=-1  OutDataTypeStr=double
  Mux : Mux  Inputs=3
  Neutral Bias : Constant  Value=[2048 2048 2048]
  Sum : Sum  Inputs=|++
  Sum1 : Sum  Inputs=|+-
  Sum2 : Sum  Inputs=|++
  Sum3 : Sum  Inputs=|++
  Processed Accel Data : Outport
  wires:
  Sum1/1 -> Gain/1
  Gain/1 -> Processed Accel Data/1
  Mux/1 -> Sum1/1
  Neutral Bias/1 -> Sum1/2
  Raw Accel Data/1 -> Data Type Conversion/1
  Demux/1 -> Gain1/1
  Sum3/1 -> Mux/1
  Demux/2 -> Gain2/1
  Gain2/1 -> Sum/1
  Sum/1 -> Mux/2
  Demux/3 -> Gain3/1
  Gain3/1 -> Sum2/1
  Sum2/1 -> Mux/3
  Bias/1 -> Sum2/2, Sum/2, Sum3/2
  Data Type Conversion/1 -> Demux/1
  Gain1/1 -> Sum3/1

== system Navigation_KF_Subsystem_child/Sensor Fusion1/Calculate Gravity Vector/Calibration_GainOffset ==
  Pre : Inport
  Accel_Calib_Gain : Constant  Value=[Accel_Calib_Gain.Gain_X Accel_Calib_Gain.Gain_Y Accel_Calib_Gain.Gain_Z]
      settings: AttributesFormatString=%<Value>
  Accel_Calib_Offset : Constant  Value="[Accel_Calib_Offset.Gain_X  Accel_Calib_Offset.Gain_Y  Accel_Calib_Offset.Gain_Z]"
      settings: AttributesFormatString=%<Value>
  Gain : Gain  Gain=-1  OutDataTypeStr=Inherit: Same as input
  Multiply : Product  Inputs=*/
  Sum : Sum  Inputs=|+-
  Post : Outport
  wires:
  Multiply/1 -> Post/1
  Accel_Calib_Offset/1 -> Sum/2
  Sum/1 -> Multiply/1
  Pre/1 -> Sum/1
  Accel_Calib_Gain/1 -> Gain/1
  Gain/1 -> Multiply/2

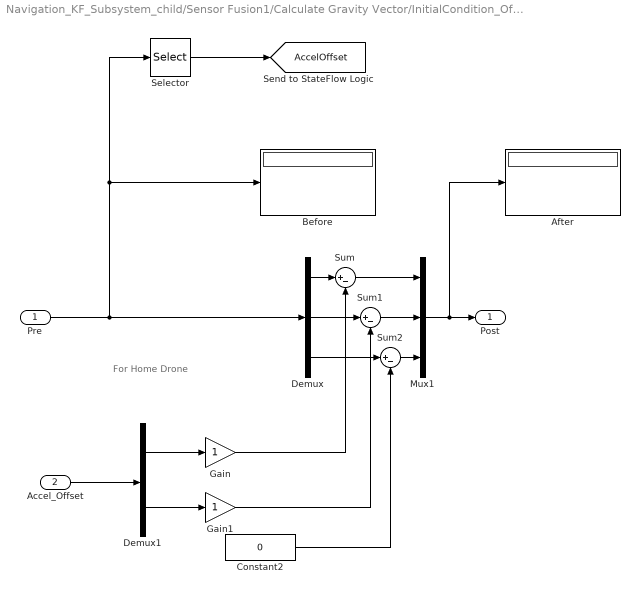
== system Navigation_KF_Subsystem_child/Sensor Fusion1/Calculate Gravity Vector/InitialCondition_Offset ==
  note: For Home Drone
  Pre : Inport
  Accel_Offset : Inport  Port=2
  After : Display
  Before : Display
  Constant2 : Constant  Value=0
  Demux : Demux  Outputs=3
  Demux1 : Demux  Outputs=2
  Gain : Gain
  Gain1 : Gain
  Mux1 : Mux  Inputs=3
  Selector : Selector  InputPortWidth=3  IndexOptions=Index vector (dialog)  Indices=[1 2]  OutputSizes=1
  Sum : Sum  Inputs=|+-
  Sum1 : Sum  Inputs=|+-
  Sum2 : Sum  Inputs=|+-
  Post : Outport
  tag scope: AccelOffset=global
  wires:
  Sum/1 -> Mux1/1
  Sum2/1 -> Mux1/3
  Demux/3 -> Sum2/1
  Sum1/1 -> Mux1/2
  Demux/1 -> Sum/1
  Demux/2 -> Sum1/1
  Mux1/1 -> Post/1, After/1
  Accel_Offset/1 -> Demux1/1
  Demux1/1 -> Gain/1
  Demux1/2 -> Gain1/1
  Pre/1 -> Demux/1, Selector/1, Before/1
  Selector/1 -> [AccelOffset]
  Gain/1 -> Sum/2
  Gain1/1 -> Sum1/2
  Constant2/1 -> Sum2/2

== system Navigation_KF_Subsystem_child/Sensor Fusion1/Calculate Gravity Vector/Low Pass Filter ==
  Offset Accel : Inport
  Add : Sum
  Gain : Gain  Gain=0.8
  Gain1 : Gain  Gain=0.2
  Unit Delay : UnitDelay  SampleTime=-1
  Filtered Accel : Outport
  wires:
  Unit Delay/1 -> Gain/1
  Gain1/1 -> Add/1
  Gain/1 -> Add/2
  Add/1 -> Unit Delay/1, Filtered Accel/1
  Offset Accel/1 -> Gain1/1

== system Navigation_KF_Subsystem_child/Sensor Fusion1/Convert/DCM to Euler Angles ==
  note: Euler Rotation Order:
      | With the camera facing towards you
      | ______________
      |       Camera          |
      | 1                    2    |
      |                             |
      | 3                    4    |
      | ______________|
      |
      | Rotation
      |
      | Roll+ , increase 2+4
      | Roll - , increase 1 3
      |
      | Pitch+ , increaes 1+2
      | Pitch- , increase 3+4
  DCM : Inport
  Constant2 : Constant  Value=[1 0 0]
  Direction Cosine Matrix to Rotation Angles : aerolibtransform2/Direction Cosine Matrix to Rotation Angles  rotationOrder=XYZ  lim=Default
      settings: AttributesFormatString=Rotation Order: %<rotationOrder>
  EulerAnglesCalculation : Subsystem  TreatAsAtomicUnit=on
  Product : Product  Multiplication=Matrix(*)
  Terminator1 : Terminator
  Terminator3 : Terminator
  Euler_Block : Outport
  wires:
  DCM/1 -> Direction Cosine Matrix to Rotation Angles/1, Product/1, EulerAnglesCalculation/1(DCM)
  Direction Cosine Matrix to Rotation Angles/1 -> Euler_Block/1
  Constant2/1 -> Product/2
  EulerAnglesCalculation/1(Euler Angles) -> Terminator3/1
  Product/1 -> Terminator1/1

== system Navigation_KF_Subsystem_child/Sensor Fusion1/KF_PITCH/Subsystem ==
  3-Axis Gyro Integrated : Inport
  Demux2 : Demux  Outputs=3
  Integrated Roll : Outport
  wires:
  Demux2/2 -> Integrated Roll/1  "Roll Axis"
  3-Axis Gyro Integrated/1 -> Demux2/1

== system Navigation_KF_Subsystem_child/Sensor Fusion1/KF_ROLL/Subsystem ==
  3-Axis Gyro Integrated : Inport
  Demux2 : Demux  Outputs=3
  Integrated Roll : Outport
  wires:
  Demux2/1 -> Integrated Roll/1  "Roll Axis"
  3-Axis Gyro Integrated/1 -> Demux2/1

== system Navigation_KF_Subsystem_child/Sensor Fusion1/Magnetometer Processing/Magnetometer Heading Calculation ==
  MagVector : Inport
  DCM : Inport  Port=2
  Compensate for Magnetic Declination (~60 degrees in Boston)_ : MATLAB Function  Commented=through  TreatAsAtomicUnit=on
  Compensate for Magnetic Declination (~67 degrees in Boston)_2 : MATLAB Function  TreatAsAtomicUnit=on
  EnlargeVectorAgain : Gain  Commented=through  Gain=3
  Transform MagVector from Body Frame to World Frame : Product  Multiplication=Matrix(*)
  Transform compensated magnetic vector into the  body frame : Product  Multiplication=Matrix(*)
  Transpose2 : Math  Operator=transpose  SaturateOnIntegerOverflow=on
  deg : Constant  Value=67
  Projected Mag Vector (body frame) : Outport
  Projected Mag Vector (global frame) : Outport  Port=2
  wires:
  MagVector/1 -> EnlargeVectorAgain/1
  Transform compensated magnetic vector into the  body frame/1 -> Projected Mag Vector (body frame)/1
  DCM/1 -> Transpose2/1, Transform MagVector from Body Frame to World Frame/1
  EnlargeVectorAgain/1 -> Transform MagVector from Body Frame to World Frame/2
  Transpose2/1 -> Transform compensated magnetic vector into the  body frame/1
  Transform MagVector from Body Frame to World Frame/1 -> Compensate for Magnetic Declination (~60 degrees in Boston)_/1(vector_in)
  Compensate for Magnetic Declination (~60 degrees in Boston)_/1(y) -> Compensate for Magnetic Declination (~67 degrees in Boston)_2/1(vector_in)
  Compensate for Magnetic Declination (~67 degrees in Boston)_2/1(y) -> Transform compensated magnetic vector into the  body frame/2, Projected Mag Vector (global frame)/1
  deg/1 -> Compensate for Magnetic Declination (~67 degrees in Boston)_2/2(declination_ang)

== system Navigation_KF_Subsystem_child/Sensor Fusion1/Magnetometer Processing/Process Raw Mag Data ==
  Magnetometer : Inport
  Process Raw Mag Data (Home_330453) : Subsystem  VariantControl=TempVariantA
  Process Raw Mag Data (Work_255725) : Subsystem  VariantControl=TempVariantB
  MagVector : Outport

== system Navigation_KF_Subsystem_child/Sensor Fusion1/Magnetometer Processing/Re-align X-axis ==
  MagVector : Inport
  Demux1 : Demux  Outputs=3
  Gain : Gain
  Gain1 : Gain  Gain=-1
  Gain2 : Gain
  Mux2 : Mux  Inputs=3
  MagVectorOut : Outport
  wires:
  Mux2/1 -> MagVectorOut/1
  Demux1/1 -> Gain1/1
  Demux1/2 -> Gain2/1
  Demux1/3 -> Gain/1
  Gain1/1 -> Mux2/1
  Gain2/1 -> Mux2/2
  Gain/1 -> Mux2/3
  MagVector/1 -> Demux1/1

== system Navigation_KF_Subsystem_child/Kalman Filter/Convert/DCM to Euler Angles/EulerAnglesCalculation ==
  DCM : Inport
  Demux : Demux  Outputs=2
  Demux1 : Demux  Outputs=2
  Gain : Gain  Gain=-1
  Gain1 : Gain  OutDataTypeStr=Inherit: Same as input
  Mux : Mux  Inputs=3
  Selector : Selector  NumberOfDimensions=2  IndexMode=Zero-based  InputPortWidth=3  IndexOptions=Index vector (dialog),Index vector (dialog)  Indices=2,0  OutputSizes=1,1
  Selector1 : Selector  NumberOfDimensions=2  IndexMode=Zero-based  InputPortWidth=3  IndexOptions=Index vector (dialog),Index vector (dialog)  Indices=2,[1 2]  OutputSizes=1,1
  Selector2 : Selector  NumberOfDimensions=2  IndexMode=Zero-based  InputPortWidth=3  IndexOptions=Index vector (dialog),Index vector (dialog)  Indices=[1 0],0  OutputSizes=1,1
  Trigonometric Function : Trigonometry  Operator=asin
  Trigonometric Function1 : Trigonometry  Operator=atan2
  Trigonometric Function2 : Trigonometry  Operator=atan2
  Euler Angles : Outport  InitialOutput=[0 0 0]
  wires:
  Demux1/2 -> Trigonometric Function2/2
  Demux1/1 -> Trigonometric Function2/1
  Mux/1 -> Euler Angles/1
  Selector2/1 -> Demux1/1  "DCM_1_0_DCM_0_0"
  Trigonometric Function2/1 -> Gain1/1  "yaw"
  Trigonometric Function1/1 -> Mux/1  "roll"
  Demux/2 -> Trigonometric Function1/2
  Demux/1 -> Trigonometric Function1/1
  Selector1/1 -> Demux/1  "DCM_2_1_DCM_2_2"
  Trigonometric Function/1 -> Mux/2  "pitch"
  Gain/1 -> Trigonometric Function/1
  Selector/1 -> Gain/1  "DCM_2_0"
  DCM/1 -> Selector/1, Selector2/1, Selector1/1
  Gain1/1 -> Mux/3

== system Navigation_KF_Subsystem_child/Sensor Fusion1/Convert/DCM to Euler Angles/EulerAnglesCalculation ==
  DCM : Inport
  Demux : Demux  Outputs=2
  Demux1 : Demux  Outputs=2
  Gain : Gain  Gain=-1
  Gain1 : Gain  OutDataTypeStr=Inherit: Same as input
  Mux : Mux  Inputs=3
  Selector : Selector  NumberOfDimensions=2  IndexMode=Zero-based  InputPortWidth=3  IndexOptions=Index vector (dialog),Index vector (dialog)  Indices=2,0  OutputSizes=1,1
  Selector1 : Selector  NumberOfDimensions=2  IndexMode=Zero-based  InputPortWidth=3  IndexOptions=Index vector (dialog),Index vector (dialog)  Indices=2,[1 2]  OutputSizes=1,1
  Selector2 : Selector  NumberOfDimensions=2  IndexMode=Zero-based  InputPortWidth=3  IndexOptions=Index vector (dialog),Index vector (dialog)  Indices=[1 0],0  OutputSizes=1,1
  Trigonometric Function : Trigonometry  Operator=asin
  Trigonometric Function1 : Trigonometry  Operator=atan2
  Trigonometric Function2 : Trigonometry  Operator=atan2
  Euler Angles : Outport  InitialOutput=[0 0 0]
  wires:
  Demux1/2 -> Trigonometric Function2/2
  Demux1/1 -> Trigonometric Function2/1
  Mux/1 -> Euler Angles/1
  Selector2/1 -> Demux1/1  "DCM_1_0_DCM_0_0"
  Trigonometric Function2/1 -> Gain1/1  "yaw"
  Trigonometric Function1/1 -> Mux/1  "roll"
  Demux/2 -> Trigonometric Function1/2
  Demux/1 -> Trigonometric Function1/1
  Selector1/1 -> Demux/1  "DCM_2_1_DCM_2_2"
  Trigonometric Function/1 -> Mux/2  "pitch"
  Gain/1 -> Trigonometric Function/1
  Selector/1 -> Gain/1  "DCM_2_0"
  DCM/1 -> Selector/1, Selector2/1, Selector1/1
  Gain1/1 -> Mux/3

== system Navigation_KF_Subsystem_child/Sensor Fusion1/Magnetometer Processing/Process Raw Mag Data/Process Raw Mag Data (Home_330453) ==
  note: magnetometer[ 0 ] = - ( float ) navdata.mx ;
      | magnetometer[ 1 ] = ( float ) navdata.my ;
      | magnetometer[ 2 ] = - ( float ) navdata.mz ;
      | const float Sensitivity[ 3 ] = { 0.0071492608 , 0.0070882491 , 0.0074057781 } ;
      | const float Neutral[ 3 ] = { 118.0 , - 65.0 , 110.0 } ;
  Magnetometer : Inport
  Bias : Constant  Commented=on  Value=[-23 4.3 1.44]
  Constant : Constant  Value=[Mag_Calib_Offset_Vector.Gain_X Mag_Calib_Offset_Vector.Gain_Y Mag_Calib_Offset_Vector.Gain_Z]
      settings: AttributesFormatString=%<Value>
  Constant1 : Constant  Value=[Mag_Calib_Gain_Vector.Gain_X Mag_Calib_Gain_Vector.Gain_Y Mag_Calib_Gain_Vector.Gain_Z]
      settings: AttributesFormatString=%<Value>
  Divide : Product  Inputs=/*
  Sum : Sum  Inputs=|+-
  postGain : Gain  Commented=on  Gain=1./[187 163 139]
  MagVector : Outport
  wires:
  Divide/1 -> MagVector/1
  Constant/1 -> Sum/2
  Magnetometer/1 -> Sum/1
  Sum/1 -> Divide/2
  Constant1/1 -> Divide/1

== system Navigation_KF_Subsystem_child/Sensor Fusion1/Magnetometer Processing/Process Raw Mag Data/Process Raw Mag Data (Work_255725) ==
  note: magnetometer[ 0 ] = - ( float ) navdata.mx ;
      | magnetometer[ 1 ] = ( float ) navdata.my ;
      | magnetometer[ 2 ] = - ( float ) navdata.mz ;
      | const float Sensitivity[ 3 ] = { 0.0071492608 , 0.0070882491 , 0.0074057781 } ;
      | const float Neutral[ 3 ] = { 118.0 , - 65.0 , 110.0 } ;
  note: 158 145 136
  Magnetometer : Inport
  Bias : Constant  Value=[2.93 18.9 77.5]
  Low Pass Filter1 : Subsystem  Commented=through
      mask Display: disp(['Elliptic Filter with 20 Hz corner', '\n', '44 dB stopband.'])
  Sum : Sum  Inputs=|+-
  postGain : Gain  Gain=1./[167 135 132]
  preGain : Gain  Commented=through  Gain=[1 1 1]
  MagVector : Outport
  wires:
  Low Pass Filter1/1(Output) -> MagVector/1
  Bias/1 -> Sum/2
  preGain/1 -> Sum/1
  Sum/1 -> postGain/1
  Magnetometer/1 -> preGain/1
  postGain/1 -> Low Pass Filter1/1(Input)

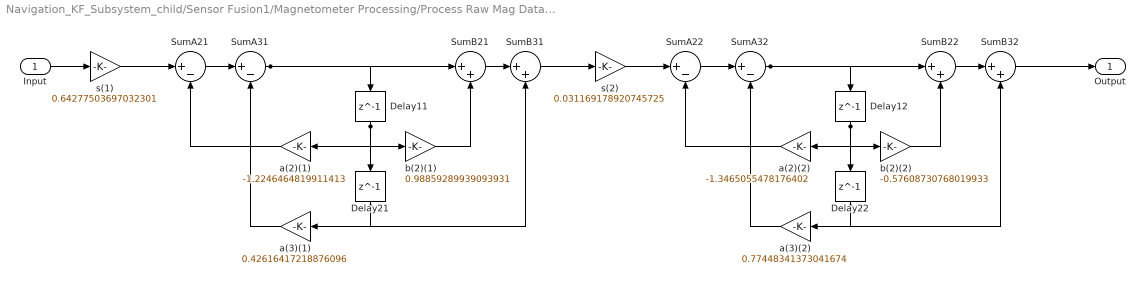
== system Navigation_KF_Subsystem_child/Sensor Fusion1/Magnetometer Processing/Process Raw Mag Data/Process Raw Mag Data (Work_255725)/Low Pass Filter1 ==
  Input : Inport
  Delay{11..12,21..22} (4 alike) : Delay  DelayLength=1  InitialCondition=0
  SumA{21..22,31..32} (4 alike) : Sum  Inputs=|+-  RndMeth=Nearest  SaturateOnIntegerOverflow=on  OutDataTypeStr=Inherit: Same as first input
  SumB{21..22,31..32} (4 alike) : Sum  Inputs=|++  RndMeth=Nearest  SaturateOnIntegerOverflow=on  OutDataTypeStr=Inherit: Same as first input
  a(2)(1) : Gain  Gain=-1.2246464819911413  ParamDataTypeStr=double  RndMeth=Nearest  SaturateOnIntegerOverflow=on  OutDataTypeStr=Inherit: Same as input
  a(2)(2) : Gain  Gain=-1.3465055478176402  ParamDataTypeStr=double  RndMeth=Nearest  SaturateOnIntegerOverflow=on  OutDataTypeStr=Inherit: Same as input
  a(3)(1) : Gain  Gain=0.42616417218876096  ParamDataTypeStr=double  RndMeth=Nearest  SaturateOnIntegerOverflow=on  OutDataTypeStr=Inherit: Same as input
  a(3)(2) : Gain  Gain=0.77448341373041674  ParamDataTypeStr=double  RndMeth=Nearest  SaturateOnIntegerOverflow=on  OutDataTypeStr=Inherit: Same as input
  b(2)(1) : Gain  Gain=0.98859289939093931  ParamDataTypeStr=double  RndMeth=Nearest  SaturateOnIntegerOverflow=on  OutDataTypeStr=Inherit: Same as input
  b(2)(2) : Gain  Gain=-0.57608730768019933  ParamDataTypeStr=double  RndMeth=Nearest  SaturateOnIntegerOverflow=on  OutDataTypeStr=Inherit: Same as input
  s(1) : Gain  Gain=0.64277503697032301  ParamDataTypeStr=double  RndMeth=Nearest  SaturateOnIntegerOverflow=on  OutDataTypeStr=Inherit: Same as input
  s(2) : Gain  Gain=0.031169178920745725  ParamDataTypeStr=double  RndMeth=Nearest  SaturateOnIntegerOverflow=on  OutDataTypeStr=Inherit: Same as input
  Output : Outport
  wires:
  Input/1 -> s(1)/1
  s(1)/1 -> SumA21/1
  SumA21/1 -> SumA31/1
  SumA31/1 -> SumB21/1, Delay11/1
  SumB21/1 -> SumB31/1
  SumB31/1 -> s(2)/1
  a(2)(1)/1 -> SumA21/2
  Delay11/1 -> a(2)(1)/1, b(2)(1)/1, Delay21/1
  b(2)(1)/1 -> SumB21/2
  a(3)(1)/1 -> SumA31/2
  Delay21/1 -> a(3)(1)/1, SumB31/2
  s(2)/1 -> SumA22/1
  SumA22/1 -> SumA32/1
  SumA32/1 -> SumB22/1, Delay12/1
  SumB22/1 -> SumB32/1
  SumB32/1 -> Output/1
  a(2)(2)/1 -> SumA22/2
  Delay12/1 -> a(2)(2)/1, b(2)(2)/1, Delay22/1
  b(2)(2)/1 -> SumB22/2
  a(3)(2)/1 -> SumA32/2
  Delay22/1 -> a(3)(2)/1, SumB32/2

== matlab function Navigation_KF_Subsystem_child/Kalman Filter/Calculate Roll - Pitch/MATLAB Function ==
  data: Ax_Ay_Az input; Roll output; Pitch output
function [Roll,Pitch] = CalculateAngle(Ax_Ay_Az)
%#codegen
Ax = -Ax_Ay_Az(1);
Ay = -Ax_Ay_Az(2);
Az = Ax_Ay_Az(3);

Pitch = atan( Ax / sqrt( Ay^2 + Az^2));
Roll = atan( Ay / sqrt( Ax^2 + Az^2));

== matlab function Navigation_KF_Subsystem_child/Sensor Fusion1/Calculate Roll - Pitch/MATLAB Function ==
  data: Ax_Ay_Az input; Roll output; Pitch output
function [Roll,Pitch] = CalculateAngle(Ax_Ay_Az)
%#codegen
Ax = -Ax_Ay_Az(1);
Ay = -Ax_Ay_Az(2);
Az = Ax_Ay_Az(3);

Pitch = atan( Ax / sqrt( Ay^2 + Az^2));
Roll = atan( Ay / sqrt( Ax^2 + Az^2));

== matlab function Navigation_KF_Subsystem_child/Sensor Fusion1/KF_PITCH/Kalman Tracker ==
  data: prev_state input; covariance_correction_prev input; state_correction output; covariance_correction output; ctrl_input_gyro input; measurement_angle input
function [state_correction, covariance_correction] = fcn(prev_state, covariance_correction_prev, ctrl_input_gyro, measurement_angle)


%-------------------------------
%-------------------------------
%---- Predict Stage ------------
%-------------------------------
%-------------------------------
% pix_value = 5;
Ts = 1/400;
%Process Noise
p_var =0.01;
Q = [p_var^2     0         
      0         p_var^2];

%A matrix
A =  [1   -Ts 
      0   1];

%odutput these values with a unit delay (for algebraic loop), apply initial conditions
state_prediction = A*prev_state + [Ts 0; 0 0]*[ctrl_input_gyro; 0 ];
covariance_prediction = A*covariance_correction_prev*A' + Q;

%-------------------------------
%-------------------------------
%---- Estimate Stage -----------
%-------------------------------
%-------------------------------

    %H matrix
    H = [1 0];

    %Measurement noise from accelerometer angle measurement
    m_var = 1;
%     m_var_r = 1;

    R = [m_var^2 ];

    %Measurement Z
    Z = [measurement_angle];

    %Compute Kalman Gain
    Kalman_Gain = covariance_prediction*H'*inv(H*covariance_prediction*H'+R); %2x2 matrix

    %compute state space correction based on measurement
    state_correction = state_prediction + Kalman_Gain*(Z - H*state_prediction); %4x1 vector of states

    %compute covariance correction
    covariance_correction = (eye(2) - Kalman_Gain*H)*covariance_prediction; %2x2 covariance matrix

%     corrected_angle_measure = state_correction(1) - Ts*state_correction(2);
end

== matlab function Navigation_KF_Subsystem_child/Sensor Fusion1/KF_ROLL/Kalman Tracker ==
  data: prev_state input; covariance_correction_prev input; state_correction output; covariance_correction output; ctrl_input_gyro input; measurement_angle input
function [state_correction, covariance_correction] = fcn(prev_state, covariance_correction_prev, ctrl_input_gyro, measurement_angle)


%-------------------------------
%-------------------------------
%---- Predict Stage ------------
%-------------------------------
%-------------------------------
% pix_value = 5;
Ts = 1/400;
%Process Noise
p_var =0.01;
Q = [p_var^2     0         
      0         p_var^2];

%A matrix
A =  [1   -Ts 
      0   1];

%odutput these values with a unit delay (for algebraic loop), apply initial conditions
state_prediction = A*prev_state + [Ts 0; 0 0]*[ctrl_input_gyro; 0 ];
covariance_prediction = A*covariance_correction_prev*A' + Q;

%-------------------------------
%-------------------------------
%---- Estimate Stage -----------
%-------------------------------
%-------------------------------

    %H matrix
    H = [1 0];

    %Measurement noise from accelerometer angle measurement
    m_var = 0.5;
%     m_var_r = 1;

    R = [m_var^2 ];

    %Measurement Z
    Z = [measurement_angle];

    %Compute Kalman Gain
    Kalman_Gain = covariance_prediction*H'*inv(H*covariance_prediction*H'+R); %2x2 matrix

    %compute state space correction based on measurement
    state_correction = state_prediction + Kalman_Gain*(Z - H*state_prediction); %4x1 vector of states

    %compute covariance correction
    covariance_correction = (eye(2) - Kalman_Gain*H)*covariance_prediction; %2x2 covariance matrix

%     corrected_angle_measure = state_correction(1) - Ts*state_correction(2);
end
